simulink model "channelizer_256"  (R2015b)
settings: Solver=FixedStepDiscrete  SolverMode=SingleTasking  StartTime=0.0  StopTime=sim_len  FixedStep=1  RelTol=1e-3
values from neighbouring files (symbols this model uses):
  N_sub = 16    [channelizer_params.m]    (also in channelizer_params_256.m = 256; channelizer_params_512.m = 512)
undefined symbols (not defined in the file or in its folder): modulator_reg_1_address, modulator_reg_1_default, modulator_reg_1_num_bits
undefined symbols (not defined in the file): reset_reg_address
libraries: xbsIndex_r4 x147
(part 2 of 2)

== system channelizer_256/channelizer/poly_phase_filter/Subsystem2 ==
  ready_in : Inport
  reset_in : Inport  Port=2
  Constant : xbsIndex_r4/Constant  const=N_sub-1  gui_display_data_type=Fixed-point  arith_type=Unsigned  n_bits=nextpow2(N_sub)  bin_pt=0  preci_type=Single  exp_width=8  frac_width=24  explicit_period=off  period=1  equ=P=C  opselect=C  inp2=PCIN>>17  opr=+  inp1=P  carry=CIN  dbl_ovrd=off  block_type=constant
  Constant1 : xbsIndex_r4/Constant  const=1  gui_display_data_type=Boolean  arith_type=Boolean  n_bits=nextpow2(N_sub)  bin_pt=0  preci_type=Single  exp_width=8  frac_width=24  explicit_period=off  period=1  equ=P=C  opselect=C  inp2=PCIN>>17  opr=+  inp1=P  carry=CIN  dbl_ovrd=off  block_type=constant
  Counter : xbsIndex_r4/Counter  cnt_type=Free Running  cnt_to=Inf  operation=Up  start_count=0  cnt_by_val=1  arith_type=Unsigned  n_bits=nextpow2(N_sub)  bin_pt=0  load_pin=off  rst=on  en=on  explicit_period=on  period=1  use_behavioral_HDL=off  implementation=Fabric  dbl_ovrd=off  block_type=counter
  Delay : xbsIndex_r4/Delay  rst=on  infoeditControl=Selection of Reset will increase slice count due to use of real FFs and instead of SRLs  en=on  latency=1  reg_retiming=off  dbl_ovrd=off  block_type=delay
  Inverter : xbsIndex_r4/Inverter  en=off  latency=0  dbl_ovrd=off  block_type=inv
  Relational : xbsIndex_r4/Relational  mode=a=b  op_type=Bool  en=off  latency=0  dbl_ovrd=off  block_type=relational
  valid_out : Outport
  last_out : Outport  Port=2
  data_out : Outport  Port=3
  wires:
  reset_in/1 -> Delay/2, Counter/1
  Counter/1 -> Relational/2, data_out/1
  Constant/1 -> Relational/1
  Relational/1 -> Delay/3, last_out/1
  ready_in/1 -> Counter/2
  Constant1/1 -> Delay/1
  Delay/1 -> Inverter/1
  Inverter/1 -> valid_out/1

== system channelizer_256/channelizer/poly_phase_filter/Subsystem3 ==
  ready : Inport
  reset_in : Inport  Port=2
  valid : Inport  Port=3
  Constant : xbsIndex_r4/Constant  const=N_sub-1  gui_display_data_type=Fixed-point  arith_type=Unsigned  n_bits=nextpow2(N_sub)  bin_pt=0  preci_type=Single  exp_width=8  frac_width=24  explicit_period=off  period=1  equ=P=C  opselect=C  inp2=PCIN>>17  opr=+  inp1=P  carry=CIN  dbl_ovrd=off  block_type=constant
  Counter : xbsIndex_r4/Counter  cnt_type=Free Running  cnt_to=Inf  operation=Up  start_count=0  cnt_by_val=1  arith_type=Unsigned  n_bits=nextpow2(N_sub)  bin_pt=0  load_pin=off  rst=on  en=on  explicit_period=on  period=1  use_behavioral_HDL=off  implementation=Fabric  dbl_ovrd=off  block_type=counter
  Logical : xbsIndex_r4/Logical  logical_function=AND  inputs=2  en=off  latency=0  precision=Full  arith_type=Unsigned  n_bits=16  bin_pt=0  align_bp=on  dbl_ovrd=off  block_type=logical
  Relational : xbsIndex_r4/Relational  mode=a=b  op_type=Bool  en=off  latency=0  dbl_ovrd=off  block_type=relational
  last_out : Outport
  wires:
  reset_in/1 -> Counter/1
  Counter/1 -> Relational/2
  Constant/1 -> Relational/1
  Relational/1 -> last_out/1
  ready/1 -> Logical/1
  valid/1 -> Logical/2
  Logical/1 -> Counter/2
